simulink model "updated_target_driver_2026_withVariants_MPC_andwlqp"  (R2024b)
settings: Solver=FixedStepDiscrete  StartTime=0.0  StopTime=running_time  FixedStep=dt_s  RelTol=1e-3
values from neighbouring files (symbols this model uses):
  A = gamma_2*gamma_3*Thrust_desired    [force2voltage.m]
  a2_lb = -0.25    [target_driver_setup_2022_Ctrl_V_2_4.m]    (also in target_driver_setup_2022_Ctrl_V_2_4_geometric.m; target_driver_setup_mpc_12msdelay.m; target_driver_setup_mpc_andWLQP.m)
  a2_openloop = 0    [target_driver_setup_2022_Ctrl_V_2_4.m]    (also in target_driver_setup_2022_Ctrl_V_2_4_geometric.m; target_driver_setup_mpc_12msdelay.m; target_driver_setup_mpc_andWLQP.m)
  a2_ub = 0.25    [target_driver_setup_2022_Ctrl_V_2_4.m]    (also in target_driver_setup_2022_Ctrl_V_2_4_geometric.m; target_driver_setup_mpc_12msdelay.m; target_driver_setup_mpc_andWLQP.m)
  att_s = 500    [target_driver_setup_2022_Ctrl_V_2_4.m]    (also in target_driver_setup_2022_Ctrl_V_2_4_geometric.m; target_driver_setup_mpc_12msdelay.m; target_driver_setup_mpc_andWLQP.m)
  b_1_d_desired = [1,0,0]    [target_driver_setup_2022_Ctrl_V_2_4.m]    (also in target_driver_setup_2022_Ctrl_V_2_4_geometric.m; target_driver_setup_mpc_12msdelay.m; target_driver_setup_mpc_andWLQP.m)
  closedloop_flag = 0    [target_driver_setup_2022_Ctrl_V_2_4.m]    (also in target_driver_setup_2022_Ctrl_V_2_4_geometric.m; target_driver_setup_mpc_12msdelay.m; target_driver_setup_mpc_andWLQP.m)
  delay = delay-vicon_sample_cycle/2    [target_driver_setup_2022_Ctrl_V_2_4.m]    (also in target_driver_setup_2022_Ctrl_V_2_4_geometric.m; target_driver_setup_mpc_12msdelay.m; target_driver_setup_mpc_andWLQP.m)
  drv_amp = abs((vleft_p2p-vright_p2p))/2+min(vleft_p2p,vright_p2p)    [Wing_traj_to_Voltage.m]    (also in force2voltage.m; target_driver_setup_2022_Ctrl_V_2_4.m = 150; target_driver_setup_2022_Ctrl_V_2_4_geometric.m = 110; target_driver_setup_mpc_12msdelay.m = 150)
  drv_bias = max_drv_bias    (= 200)    [target_driver_setup_2022_Ctrl_V_2_4.m]    (also in target_driver_setup_2022_Ctrl_V_2_4_geometric.m; target_driver_setup_mpc_12msdelay.m; target_driver_setup_mpc_andWLQP.m)
  drv_pitch_left = vleft_pitch    [Wing_traj_to_Voltage.m]    (also in force2voltage.m = 0; target_driver_setup_2022_Ctrl_V_2_4.m = 9.05; target_driver_setup_2022_Ctrl_V_2_4_geometric.m = 9.05; target_driver_setup_mpc_12msdelay.m = 9.05)
  drv_pitch_right = vright_pitch    [Wing_traj_to_Voltage.m]    (also in force2voltage.m = 0; target_driver_setup_2022_Ctrl_V_2_4.m = 9.05; target_driver_setup_2022_Ctrl_V_2_4_geometric.m = 9.05; target_driver_setup_mpc_12msdelay.m = 9.05)
  drv_roll = (vleft_p2p-vright_p2p)/4    [Wing_traj_to_Voltage.m]    (also in force2voltage.m; target_driver_setup_2022_Ctrl_V_2_4.m = -0.001; target_driver_setup_2022_Ctrl_V_2_4_geometric.m = -0.001; target_driver_setup_mpc_12msdelay.m = -0.001)
  dt_s = 2.0e-4    (= 0.0002)    [target_driver_setup_2022_Ctrl_V_2_4.m]    (also in target_driver_setup_2022_Ctrl_V_2_4_geometric.m; target_driver_setup_mpc_12msdelay.m; target_driver_setup_mpc_andWLQP.m)
  f_fin = f    (= 155)    [target_driver_setup_2022_Ctrl_V_2_4.m]    (also in target_driver_setup_2022_Ctrl_V_2_4_geometric.m; target_driver_setup_mpc_12msdelay.m; target_driver_setup_mpc_andWLQP.m)
  f_int = f    (= 155)    [target_driver_setup_2022_Ctrl_V_2_4.m]    (also in target_driver_setup_2022_Ctrl_V_2_4_geometric.m; target_driver_setup_mpc_12msdelay.m; target_driver_setup_mpc_andWLQP.m)
  g = 9.8    [target_driver_setup_2022_Ctrl_V_2_4.m]    (also in target_driver_setup_2022_Ctrl_V_2_4_geometric.m; target_driver_setup_mpc_12msdelay.m; target_driver_setup_mpc_andWLQP.m; test_full_attitude_mpc.m = 9.81)
  I_moment_vec = [Ixx, Iyy, Izz]    [target_driver_setup_2022_Ctrl_V_2_4.m]    (also in target_driver_setup_2022_Ctrl_V_2_4_geometric.m; target_driver_setup_mpc_12msdelay.m; target_driver_setup_mpc_andWLQP.m)
  k_tau_vec = [k_tau_roll;k_tau_pitch]    [target_driver_setup_2022_Ctrl_V_2_4.m]    (also in target_driver_setup_2022_Ctrl_V_2_4_geometric.m; target_driver_setup_mpc_12msdelay.m; target_driver_setup_mpc_andWLQP.m)
  landing_flag = 0    [target_driver_setup_2022_Ctrl_V_2_4.m]    (also in target_driver_setup_2022_Ctrl_V_2_4_geometric.m; target_driver_setup_mpc_12msdelay.m; target_driver_setup_mpc_andWLQP.m)
  landing_parameter = [start_delay+T,transition_rate, rising_time, falling_time, landing_rising_time, landing_z_decrease, landing_y_decrease, landing_x_decrease]    [target_driver_setup_2022_Ctrl_V_2_4.m]    (also in target_driver_setup_2022_Ctrl_V_2_4_geometric.m; target_driver_setup_mpc_12msdelay.m; target_driver_setup_mpc_andWLQP.m)
  low_bound = -5    [target_driver_setup_2022_Ctrl_V_2_4.m]    (also in target_driver_setup_2022_Ctrl_V_2_4_geometric.m; target_driver_setup_mpc_12msdelay.m = -10; target_driver_setup_mpc_andWLQP.m = -10)
  low_bound_eR = -1.2    [target_driver_setup_2022_Ctrl_V_2_4.m]    (also in target_driver_setup_2022_Ctrl_V_2_4_geometric.m; target_driver_setup_mpc_12msdelay.m; target_driver_setup_mpc_andWLQP.m)
  low_bound_vx = -0.5    [target_driver_setup_2022_Ctrl_V_2_4.m]    (also in target_driver_setup_2022_Ctrl_V_2_4_geometric.m; target_driver_setup_mpc_12msdelay.m; target_driver_setup_mpc_andWLQP.m)
  low_bound_vy = -0.5    [target_driver_setup_2022_Ctrl_V_2_4.m]    (also in target_driver_setup_2022_Ctrl_V_2_4_geometric.m; target_driver_setup_mpc_12msdelay.m; target_driver_setup_mpc_andWLQP.m)
  low_bound_vz = -0.5    [target_driver_setup_2022_Ctrl_V_2_4.m]    (also in target_driver_setup_2022_Ctrl_V_2_4_geometric.m; target_driver_setup_mpc_12msdelay.m; target_driver_setup_mpc_andWLQP.m)
  low_bound_x = -0.1    [target_driver_setup_2022_Ctrl_V_2_4.m]    (also in target_driver_setup_2022_Ctrl_V_2_4_geometric.m; target_driver_setup_mpc_12msdelay.m = -0.6; target_driver_setup_mpc_andWLQP.m = -0.6)
  low_bound_y = -0.06    [target_driver_setup_2022_Ctrl_V_2_4.m]    (also in target_driver_setup_2022_Ctrl_V_2_4_geometric.m; target_driver_setup_mpc_12msdelay.m = -0.6; target_driver_setup_mpc_andWLQP.m = -0.6)
  low_bound_z = -0.04    [target_driver_setup_2022_Ctrl_V_2_4.m]    (also in target_driver_setup_2022_Ctrl_V_2_4_geometric.m; target_driver_setup_mpc_12msdelay.m = -0.1; target_driver_setup_mpc_andWLQP.m = -0.1)
  m = t <= t_zoom    [plot_roll_torque_cmd_vs_actual.m]    (also in plot_roll_torque_cmd_vs_actual_flightlog.m = t >= t0 & t <= t1; target_driver_setup_2022_Ctrl_V_2_4.m = 8.5655e-05; target_driver_setup_2022_Ctrl_V_2_4_geometric.m = 8.5655e-05; target_driver_setup_mpc_12msdelay.m = 8.5655e-05)
  params_vec = [params_opt.delta_1, params_opt.delta_2, params_opt.delta_3,      params_opt.gamma_1, params_opt.gamma_2_1, params_opt.gamma_3,      params_opt.eta, params_opt.nu, params_opt.mu]'    [force2voltage_tuningSandbox.m]    (also in target_driver_setup_2022_Ctrl_V_2_4.m = [params_opt.delta_1, params_opt.delta_2, params_opt.delta_3,; target_driver_setup_2022_Ctrl_V_2_4_geometric.m = [params_opt.delta_1, params_opt.delta_2, params_opt.delta_3,; target_driver_setup_mpc_12msdelay.m = [params_opt.delta_1, params_opt.delta_2, params_opt.delta_3,; target_driver_setup_mpc_andWLQP.m = [params_opt.delta_1, params_opt.delta_2, params_opt.delta_3,)
  phase = 0    [target_driver_setup_2022_Ctrl_V_2_4.m]    (also in target_driver_setup_2022_Ctrl_V_2_4_geometric.m; target_driver_setup_mpc_12msdelay.m; target_driver_setup_mpc_andWLQP.m)
  r_desired = [default_x, default_y,z_desired]    [target_driver_setup_2022_Ctrl_V_2_4.m]    (also in target_driver_setup_2022_Ctrl_V_2_4_geometric.m; target_driver_setup_mpc_12msdelay.m; target_driver_setup_mpc_andWLQP.m)
  roll_offset_angle = 0    [target_driver_setup_2022_Ctrl_V_2_4.m]    (also in target_driver_setup_2022_Ctrl_V_2_4_geometric.m; target_driver_setup_mpc_12msdelay.m; target_driver_setup_mpc_andWLQP.m)
  running_time = start_delay+T    (= 10)    [target_driver_setup_2022_Ctrl_V_2_4.m]    (also in target_driver_setup_2022_Ctrl_V_2_4_geometric.m; target_driver_setup_mpc_12msdelay.m = 0.5; target_driver_setup_mpc_andWLQP.m)
  running_time_control = start_delay_control+T+0.0    (= 10)    [target_driver_setup_2022_Ctrl_V_2_4.m]    (also in target_driver_setup_2022_Ctrl_V_2_4_geometric.m; target_driver_setup_mpc_12msdelay.m = 0.5; target_driver_setup_mpc_andWLQP.m)
  sampling_f = 1/dt_s    (= 5000)    [target_driver_setup_2022_Ctrl_V_2_4.m]    (also in target_driver_setup_2022_Ctrl_V_2_4_geometric.m; target_driver_setup_mpc_12msdelay.m; target_driver_setup_mpc_andWLQP.m)
  start_delay = 0.0    (= 0)    [target_driver_setup_2022_Ctrl_V_2_4.m]    (also in target_driver_setup_2022_Ctrl_V_2_4_geometric.m; target_driver_setup_mpc_12msdelay.m; target_driver_setup_mpc_andWLQP.m)
  start_delay_control = start_delay + ramp_delay    (= 0)    [target_driver_setup_2022_Ctrl_V_2_4.m]    (also in target_driver_setup_2022_Ctrl_V_2_4_geometric.m; target_driver_setup_mpc_12msdelay.m; target_driver_setup_mpc_andWLQP.m)
  T = 10    [target_driver_setup_2022_Ctrl_V_2_4.m]    (also in target_driver_setup_2022_Ctrl_V_2_4_geometric.m; target_driver_setup_mpc_12msdelay.m = 0.5; target_driver_setup_mpc_andWLQP.m; test_full_attitude_mpc.m = T0 + nu(1))
  task_flag = 0    [target_driver_setup_2022_Ctrl_V_2_4.m]    (also in target_driver_setup_2022_Ctrl_V_2_4_geometric.m; target_driver_setup_mpc_12msdelay.m; target_driver_setup_mpc_andWLQP.m)
  task_parameter = [radius_ref, frequency_ref, radius_ratio, lissajous_ratio, lissajous_delta, lissajous_amplitude_ratio,z_radius_ratio]    [target_driver_setup_2022_Ctrl_V_2_4.m]    (also in target_driver_setup_2022_Ctrl_V_2_4_geometric.m; target_driver_setup_mpc_12msdelay.m; target_driver_setup_mpc_andWLQP.m)
  upp_bound = 5    [target_driver_setup_2022_Ctrl_V_2_4.m]    (also in target_driver_setup_2022_Ctrl_V_2_4_geometric.m; target_driver_setup_mpc_12msdelay.m = 10; target_driver_setup_mpc_andWLQP.m = 10)
  upp_bound_eR = 1.2    [target_driver_setup_2022_Ctrl_V_2_4.m]    (also in target_driver_setup_2022_Ctrl_V_2_4_geometric.m; target_driver_setup_mpc_12msdelay.m; target_driver_setup_mpc_andWLQP.m)
  upp_bound_vx = 0.5    [target_driver_setup_2022_Ctrl_V_2_4.m]    (also in target_driver_setup_2022_Ctrl_V_2_4_geometric.m; target_driver_setup_mpc_12msdelay.m; target_driver_setup_mpc_andWLQP.m)
  upp_bound_vy = 0.5    [target_driver_setup_2022_Ctrl_V_2_4.m]    (also in target_driver_setup_2022_Ctrl_V_2_4_geometric.m; target_driver_setup_mpc_12msdelay.m; target_driver_setup_mpc_andWLQP.m)
  upp_bound_vz = 0.5    [target_driver_setup_2022_Ctrl_V_2_4.m]    (also in target_driver_setup_2022_Ctrl_V_2_4_geometric.m; target_driver_setup_mpc_12msdelay.m; target_driver_setup_mpc_andWLQP.m)
  upp_bound_x = 0.1    [target_driver_setup_2022_Ctrl_V_2_4.m]    (also in target_driver_setup_2022_Ctrl_V_2_4_geometric.m; target_driver_setup_mpc_12msdelay.m = 0.6; target_driver_setup_mpc_andWLQP.m = 0.6)
  upp_bound_y = 0.06    [target_driver_setup_2022_Ctrl_V_2_4.m]    (also in target_driver_setup_2022_Ctrl_V_2_4_geometric.m; target_driver_setup_mpc_12msdelay.m = 0.6; target_driver_setup_mpc_andWLQP.m = 0.6)
  upp_bound_z = 0.04    [target_driver_setup_2022_Ctrl_V_2_4.m]    (also in target_driver_setup_2022_Ctrl_V_2_4_geometric.m; target_driver_setup_mpc_12msdelay.m = 0.1; target_driver_setup_mpc_andWLQP.m = 0.1)
  weights_vec = [ws; wds; wpr_xy;wpr_z; wpf; wvr_xy; wvr_z ... (first row only)    [target_driver_setup_2022_Ctrl_V_2_4.m]    (also in target_driver_setup_2022_Ctrl_V_2_4_geometric.m; target_driver_setup_mpc_12msdelay.m; target_driver_setup_mpc_andWLQP.m)
undefined symbols (not defined in the file or in its folder): Com1, ctrl_Ts, DiscIntNeverNeededParam, dspblkCoreblockFVToolHelper, gcbh, left_mapping, left_mapping_F_to_Phi, lp_den, lp_num, none, right_mapping, right_mapping_F_to_Phi, vlp_den, vlp_num
libraries: simulink x18, xpcseriallib x2, cstblocks x1, xpcnilib x1, xpcutilitieslib x1
(part 3 of 6)

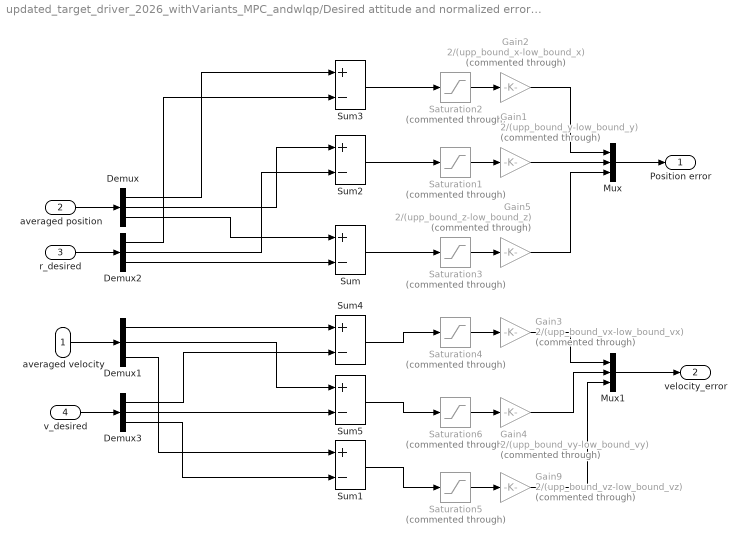
== system updated_target_driver_2026_withVariants_MPC_andwlqp/Desired attitude and normalized error/Variant Subsystem/unsaturated normalized error observation1/saturated normalized altitude error  ==
  averaged velocity : Inport
  averaged position : Inport  Port=2
  "r_desired " : Inport  Port=3
  v_desired : Inport  Port=4
  Demux{,1..3} (4 alike) : Demux  Outputs=3
  Gain1 : Gain  Commented=through  Gain=2/(upp_bound_y-low_bound_y)
  Gain2 : Gain  Commented=through  Gain=2/(upp_bound_x-low_bound_x)
  Gain3 : Gain  Commented=through  Gain=2/(upp_bound_vx-low_bound_vx)
  Gain4 : Gain  Commented=through  Gain=2/(upp_bound_vy-low_bound_vy)
  Gain5 : Gain  Commented=through  Gain=2/(upp_bound_z-low_bound_z)
  Gain9 : Gain  Commented=through  Gain=2/(upp_bound_vz-low_bound_vz)
  Mux : Mux  Inputs=3
  Mux1 : Mux  Inputs=3
  Saturation1 : Saturate  Commented=through  UpperLimit=upp_bound_y  LowerLimit=low_bound_y
  Saturation2 : Saturate  Commented=through  UpperLimit=upp_bound_x  LowerLimit=low_bound_x
  Saturation3 : Saturate  Commented=through  UpperLimit=upp_bound_z  LowerLimit=low_bound_z
  Saturation4 : Saturate  Commented=through  UpperLimit=upp_bound_vx  LowerLimit=low_bound_vx
  Saturation5 : Saturate  Commented=through  UpperLimit=upp_bound_vz  LowerLimit=low_bound_vz
  Saturation6 : Saturate  Commented=through  UpperLimit=upp_bound_vy  LowerLimit=low_bound_vy
  Sum{,1..5} (6 alike) : Sum  Inputs=+-
  Position error : Outport
  velocity_error : Outport  Port=2
  wires:
  Demux2/3 -> Sum/2
  Sum/1 -> Saturation3/1
  Sum1/1 -> Saturation5/1
  Gain5/1 -> Mux/3
  Saturation3/1 -> Gain5/1
  Saturation5/1 -> Gain9/1
  Gain9/1 -> Mux1/3
  Mux1/1 -> velocity_error/1
  averaged velocity/1 -> Demux1/1
  averaged position/1 -> Demux/1
  Demux/3 -> Sum/1
  Demux1/3 -> Sum1/1
  "r_desired "/1 -> Demux2/1
  Saturation1/1 -> Gain1/1
  Sum2/1 -> Saturation1/1
  Demux2/2 -> Sum2/2
  Demux/2 -> Sum2/1
  Sum3/1 -> Saturation2/1
  Saturation2/1 -> Gain2/1
  Demux/1 -> Sum3/1
  Demux2/1 -> Sum3/2
  v_desired/1 -> Demux3/1
  Demux3/3 -> Sum1/2
  Saturation4/1 -> Gain3/1
  Gain3/1 -> Mux1/1
  Sum4/1 -> Saturation4/1
  Demux3/1 -> Sum4/2
  Demux1/1 -> Sum4/1
  Saturation6/1 -> Gain4/1
  Gain4/1 -> Mux1/2
  Sum5/1 -> Saturation6/1
  Demux3/2 -> Sum5/2
  Demux1/2 -> Sum5/1
  Gain2/1 -> Mux/1
  Gain1/1 -> Mux/2
  Mux/1 -> Position error/1

== system updated_target_driver_2026_withVariants_MPC_andwlqp/Observer for averaged system1/Attitude Observer/Geometric Averaging Rotation Matix/Geometric Averaging Rotation M ==
  "Current Rotation " : Inport
  Vicon Update : Inport  Port=2
  "Previous Averaged Rotation " : Inport  Port=3
  Delay1 : Delay  DelayLength=delay(5)  InitialCondition=0
  Delay3 : Delay  DelayLength=delay(2)  InitialCondition=0
  Delay4 : Delay  DelayLength=delay(3)  InitialCondition=0
  Delay5 : Delay  DelayLength=delay(4)  InitialCondition=0
  Delay7 : Delay  DelayLength=delay(6)  InitialCondition=0
  Delay9 : Delay  DelayLength=delay(7)  InitialCondition=0
  "Geometric Average " : MATLAB Function  TreatAsAtomicUnit=on
  Averaged Rotation Matrix : Outport
  wires:
  Delay5/1 -> "Geometric Average "/3(R_prev3)
  Delay4/1 -> "Geometric Average "/2(R_prev2)
  "Geometric Average "/1(Rout) -> Averaged Rotation Matrix/1
  Delay3/1 -> "Geometric Average "/1(R_prev)
  Delay9/1 -> "Geometric Average "/6(R_prev6)
  Delay7/1 -> "Geometric Average "/5(R_prev5)
  Delay1/1 -> "Geometric Average "/4(R_prev4)
  Vicon Update/1 -> "Geometric Average "/8(update)
  "Current Rotation "/1 -> "Geometric Average "/7(R_cur), Delay9/1, Delay7/1, Delay1/1, Delay5/1, Delay4/1, Delay3/1
  "Previous Averaged Rotation "/1 -> "Geometric Average "/9(Rout_prev)

== system updated_target_driver_2026_withVariants_MPC_andwlqp/Observer for averaged system1/Attitude Observer/Geometric derivative in SO(3)/filtered derivative5 ==
  In1 : Inport
  low pass3 : DiscreteTransferFcn  Numerator=lp_num  Denominator=lp_den
  Out1 : Outport
  wires:
  low pass3/1 -> Out1/1
  In1/1 -> low pass3/1

== system updated_target_driver_2026_withVariants_MPC_andwlqp/Variant Subsystem/Experimental/signal generator a3/Bias_Signal ==
  note: time constant = 0.002sec
  QuasiEnable : Inport
  BiasVolts : Inport  Port=2
  AveragedBias : Subsystem
  PreGain : Gain
  Product : Product  RndMeth=Zero
  SIgnalForRamp_binary : Subsystem
  SaturatingRamp : DiscreteIntegrator  gainval=10  SampleTime=-1  LimitOutput=on  UpperSaturationLimit=1  LowerSaturationLimit=0  ICPrevOutput=DiscIntNeverNeededParam  ICPrevScaledInput=DiscIntNeverNeededParam
  BiasD2A : Outport
  wires:
  PreGain/1 -> BiasD2A/1
  BiasVolts/1 -> AveragedBias/1(In1)
  QuasiEnable/1 -> SIgnalForRamp_binary/1(In1)
  SIgnalForRamp_binary/1(Out1) -> SaturatingRamp/1
  SaturatingRamp/1 -> Product/1
  AveragedBias/1(Out1) -> Product/2
  Product/1 -> PreGain/1

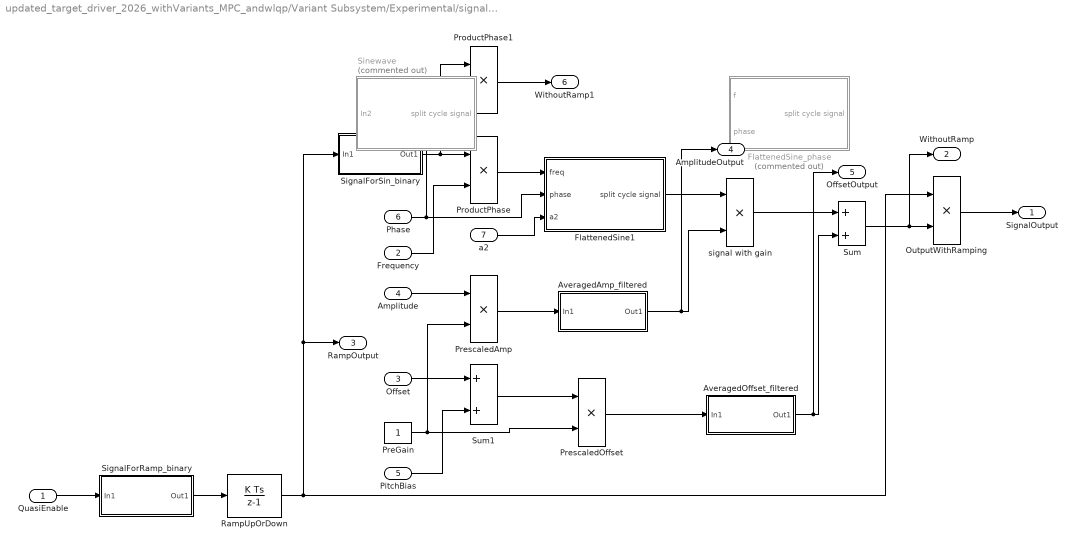
== system updated_target_driver_2026_withVariants_MPC_andwlqp/Variant Subsystem/Experimental/signal generator a3/Drive_Signal ==
  QuasiEnable : Inport
  Frequency : Inport  Port=2
  Offset : Inport  Port=3
  Amplitude : Inport  Port=4
  PitchBias : Inport  Port=5
  Phase : Inport  Port=6
  "a2 " : Inport  Port=7
  AveragedAmp_filtered : Subsystem
  AveragedOffset_filtered : Subsystem
  FlattenedSine1 : Subsystem
  FlattenedSine_phase : Subsystem  Commented=on
  OutputWithRamping : Product  RndMeth=Zero
  PreGain : Constant
  PrescaledAmp : Product  RndMeth=Zero
  PrescaledOffset : Product  RndMeth=Zero
  ProductPhase : Product  RndMeth=Zero
  ProductPhase1 : Product  RndMeth=Zero
  RampUpOrDown : DiscreteIntegrator  gainval=10  SampleTime=-1  LimitOutput=on  UpperSaturationLimit=1  LowerSaturationLimit=0  ICPrevOutput=DiscIntNeverNeededParam  ICPrevScaledInput=DiscIntNeverNeededParam
  SignalForRamp_binary : Subsystem
  SignalForSin_binary : Subsystem
  Sinewave : Subsystem  Commented=on
  Sum : Sum
  Sum1 : Sum
  signal with gain : Product  RndMeth=Zero
  SignalOutput : Outport
  WithoutRamp : Outport  Port=2
  RampOutput : Outport  Port=3
  AmplitudeOutput : Outport  Port=4
  OffsetOutput : Outport  Port=5
  WithoutRamp1 : Outport  Port=6
  wires:
  OutputWithRamping/1 -> SignalOutput/1
  Sum/1 -> WithoutRamp/1, OutputWithRamping/2
  PrescaledOffset/1 -> AveragedOffset_filtered/1(In1)
  AveragedAmp_filtered/1(Out1) -> AmplitudeOutput/1, signal with gain/2
  PrescaledAmp/1 -> AveragedAmp_filtered/1(In1)
  "a2 "/1 -> FlattenedSine1/3(a2)
  ProductPhase/1 -> FlattenedSine1/1(freq)
  ProductPhase1/1 -> WithoutRamp1/1
  Offset/1 -> Sum1/1
  AveragedOffset_filtered/1(Out1) -> OffsetOutput/1, Sum/2
  signal with gain/1 -> Sum/1
  SignalForSin_binary/1(Out1) -> ProductPhase1/1, ProductPhase/1
  Amplitude/1 -> PrescaledAmp/1
  Sum1/1 -> PrescaledOffset/1
  Frequency/1 -> ProductPhase/2
  PreGain/1 -> PrescaledAmp/2, PrescaledOffset/2
  FlattenedSine1/1(split cycle signal) -> signal with gain/1
  QuasiEnable/1 -> SignalForRamp_binary/1(In1)
  SignalForRamp_binary/1(Out1) -> RampUpOrDown/1
  Phase/1 -> ProductPhase1/2, FlattenedSine1/2(phase)
  PitchBias/1 -> Sum1/2
  RampUpOrDown/1 -> SignalForSin_binary/1(In1), RampOutput/1, OutputWithRamping/1

== system updated_target_driver_2026_withVariants_MPC_andwlqp/Variant Subsystem/Experimental/signal generator a3/Drive_Signal1 ==
  QuasiEnable : Inport
  Frequency : Inport  Port=2
  Offset : Inport  Port=3
  Amplitude : Inport  Port=4
  PitchBias : Inport  Port=5
  a2 : Inport  Port=6
  AveragedAmp_filtered : Subsystem
  AveragedOffset_filtered : Subsystem
  FlattenedSine1 : Subsystem
  OutputWithRamping : Product  RndMeth=Zero
  PreGain : Constant
  PrescaledAmp : Product  RndMeth=Zero
  PrescaledOffset : Product  RndMeth=Zero
  ProductPhase : Product  RndMeth=Zero
  RampUpOrDown : DiscreteIntegrator  gainval=10  SampleTime=-1  LimitOutput=on  UpperSaturationLimit=1  LowerSaturationLimit=0  ICPrevOutput=DiscIntNeverNeededParam  ICPrevScaledInput=DiscIntNeverNeededParam
  SignalForRamp_binary : Subsystem
  SignalForSin_binary : Subsystem
  Sine Wave : Subsystem  Commented=on
  Sum : Sum
  Sum1 : Sum
  signal with gain : Product  RndMeth=Zero
  SignalOutput : Outport
  WithoutRamp : Outport  Port=2
  RampOutput : Outport  Port=3
  AmplitudeOutput : Outport  Port=4
  OffsetOutput : Outport  Port=5
  wires:
  PrescaledAmp/1 -> AveragedAmp_filtered/1(In1)
  Sum/1 -> OutputWithRamping/2, WithoutRamp/1
  RampUpOrDown/1 -> RampOutput/1, OutputWithRamping/1, SignalForSin_binary/1(In1)
  QuasiEnable/1 -> SignalForRamp_binary/1(In1)
  SignalForRamp_binary/1(Out1) -> RampUpOrDown/1
  signal with gain/1 -> Sum/1
  Frequency/1 -> ProductPhase/2
  SignalForSin_binary/1(Out1) -> ProductPhase/1
  AveragedOffset_filtered/1(Out1) -> Sum/2, OffsetOutput/1
  PrescaledOffset/1 -> AveragedOffset_filtered/1(In1)
  PreGain/1 -> PrescaledAmp/2, PrescaledOffset/2
  OutputWithRamping/1 -> SignalOutput/1
  AveragedAmp_filtered/1(Out1) -> signal with gain/2, AmplitudeOutput/1
  Sum1/1 -> PrescaledOffset/1
  Offset/1 -> Sum1/1
  PitchBias/1 -> Sum1/2
  Amplitude/1 -> PrescaledAmp/1
  ProductPhase/1 -> FlattenedSine1/1(freq)
  FlattenedSine1/1(split cycle signal) -> signal with gain/1
  a2/1 -> FlattenedSine1/2(a2)

== system updated_target_driver_2026_withVariants_MPC_andwlqp/Variant Subsystem/Experimental/signal generator a3/SignalSaturationLimit ==
  BiasMax : Inport
  SignalRaw : Inport  Port=2
  GainBias : Gain
  MaxOf : MinMax  Function=max  Inputs=2
  MinOf : MinMax  Inputs=2
  ground : Constant
  SignalSatd : Outport
  wires:
  BiasMax/1 -> GainBias/1
  SignalRaw/1 -> MinOf/2
  MinOf/1 -> MaxOf/1
  MaxOf/1 -> SignalSatd/1
  GainBias/1 -> MinOf/1
  ground/1 -> MaxOf/2

== system updated_target_driver_2026_withVariants_MPC_andwlqp/Variant Subsystem/Experimental/signal generator a3/SignalSaturationLimit1 ==
  BiasMax : Inport
  SignalRaw : Inport  Port=2
  GainBias : Gain
  MaxOf : MinMax  Function=max  Inputs=2
  MinOf : MinMax  Inputs=2
  ground : Constant
  SignalSatd : Outport
  wires:
  BiasMax/1 -> GainBias/1
  SignalRaw/1 -> MinOf/2
  MinOf/1 -> MaxOf/1
  MaxOf/1 -> SignalSatd/1
  GainBias/1 -> MinOf/1
  ground/1 -> MaxOf/2

== system updated_target_driver_2026_withVariants_MPC_andwlqp/Variant Subsystem/Simulation/signal generator a3/Bias_Signal ==
  note: time constant = 0.002sec
  QuasiEnable : Inport
  BiasVolts : Inport  Port=2
  AveragedBias : Subsystem
  PreGain : Gain
  Product : Product  RndMeth=Zero
  SIgnalForRamp_binary : Subsystem
  SaturatingRamp : DiscreteIntegrator  Commented=through  gainval=10  SampleTime=-1  LimitOutput=on  UpperSaturationLimit=1  LowerSaturationLimit=0  ICPrevOutput=DiscIntNeverNeededParam  ICPrevScaledInput=DiscIntNeverNeededParam
  BiasD2A : Outport
  wires:
  PreGain/1 -> BiasD2A/1
  BiasVolts/1 -> AveragedBias/1(In1)
  QuasiEnable/1 -> SIgnalForRamp_binary/1(In1)
  SIgnalForRamp_binary/1(Out1) -> SaturatingRamp/1
  SaturatingRamp/1 -> Product/1
  AveragedBias/1(Out1) -> Product/2
  Product/1 -> PreGain/1

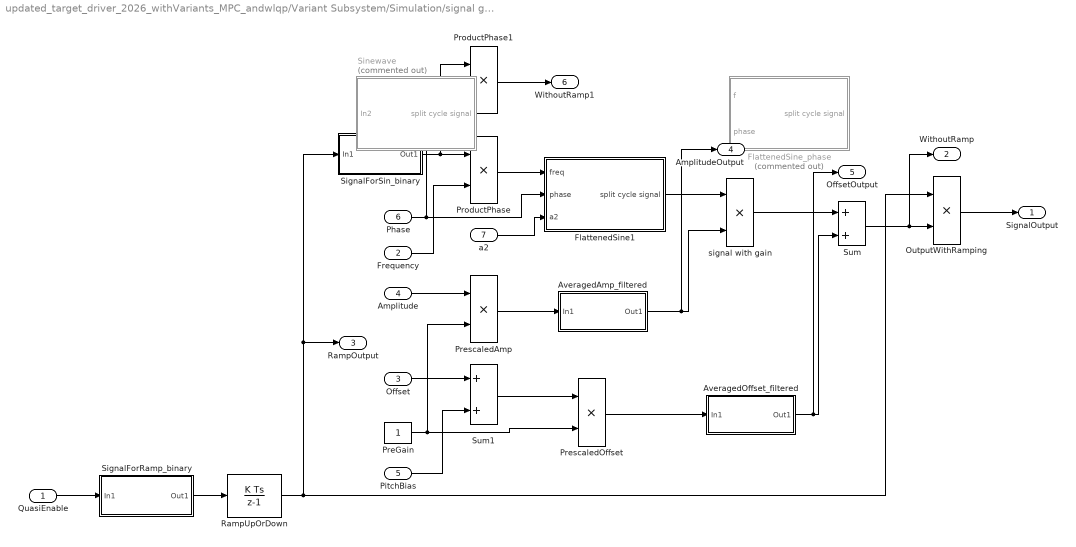
== system updated_target_driver_2026_withVariants_MPC_andwlqp/Variant Subsystem/Simulation/signal generator a3/Drive_Signal ==
  QuasiEnable : Inport
  Frequency : Inport  Port=2
  Offset : Inport  Port=3
  Amplitude : Inport  Port=4
  PitchBias : Inport  Port=5
  Phase : Inport  Port=6
  "a2 " : Inport  Port=7
  AveragedAmp_filtered : Subsystem
  AveragedOffset_filtered : Subsystem
  FlattenedSine1 : Subsystem
  FlattenedSine_phase : Subsystem  Commented=on
  OutputWithRamping : Product  RndMeth=Zero
  PreGain : Constant
  PrescaledAmp : Product  RndMeth=Zero
  PrescaledOffset : Product  RndMeth=Zero
  ProductPhase : Product  RndMeth=Zero
  ProductPhase1 : Product  RndMeth=Zero
  RampUpOrDown : DiscreteIntegrator  gainval=10  SampleTime=-1  LimitOutput=on  UpperSaturationLimit=1  LowerSaturationLimit=0  ICPrevOutput=DiscIntNeverNeededParam  ICPrevScaledInput=DiscIntNeverNeededParam
  SignalForRamp_binary : Subsystem
  SignalForSin_binary : Subsystem
  Sinewave : Subsystem  Commented=on
  Sum : Sum
  Sum1 : Sum
  signal with gain : Product  RndMeth=Zero
  SignalOutput : Outport
  WithoutRamp : Outport  Port=2
  RampOutput : Outport  Port=3
  AmplitudeOutput : Outport  Port=4
  OffsetOutput : Outport  Port=5
  WithoutRamp1 : Outport  Port=6
  wires:
  OutputWithRamping/1 -> SignalOutput/1
  Sum/1 -> WithoutRamp/1, OutputWithRamping/2
  PrescaledOffset/1 -> AveragedOffset_filtered/1(In1)
  AveragedAmp_filtered/1(Out1) -> AmplitudeOutput/1, signal with gain/2
  PrescaledAmp/1 -> AveragedAmp_filtered/1(In1)
  "a2 "/1 -> FlattenedSine1/3(a2)
  ProductPhase/1 -> FlattenedSine1/1(freq)
  ProductPhase1/1 -> WithoutRamp1/1
  Offset/1 -> Sum1/1
  AveragedOffset_filtered/1(Out1) -> OffsetOutput/1, Sum/2
  signal with gain/1 -> Sum/1
  SignalForSin_binary/1(Out1) -> ProductPhase1/1, ProductPhase/1
  Amplitude/1 -> PrescaledAmp/1
  Sum1/1 -> PrescaledOffset/1
  Frequency/1 -> ProductPhase/2
  PreGain/1 -> PrescaledAmp/2, PrescaledOffset/2
  FlattenedSine1/1(split cycle signal) -> signal with gain/1
  QuasiEnable/1 -> SignalForRamp_binary/1(In1)
  SignalForRamp_binary/1(Out1) -> RampUpOrDown/1
  Phase/1 -> ProductPhase1/2, FlattenedSine1/2(phase)
  PitchBias/1 -> Sum1/2
  RampUpOrDown/1 -> SignalForSin_binary/1(In1), RampOutput/1, OutputWithRamping/1

== system updated_target_driver_2026_withVariants_MPC_andwlqp/Variant Subsystem/Simulation/signal generator a3/Drive_Signal1 ==
  QuasiEnable : Inport
  Frequency : Inport  Port=2
  Offset : Inport  Port=3
  Amplitude : Inport  Port=4
  PitchBias : Inport  Port=5
  a2 : Inport  Port=6
  AveragedAmp_filtered : Subsystem
  AveragedOffset_filtered : Subsystem
  FlattenedSine1 : Subsystem
  OutputWithRamping : Product  RndMeth=Zero
  PreGain : Constant
  PrescaledAmp : Product  RndMeth=Zero
  PrescaledOffset : Product  RndMeth=Zero
  ProductPhase : Product  RndMeth=Zero
  RampUpOrDown : DiscreteIntegrator  gainval=10  SampleTime=-1  LimitOutput=on  UpperSaturationLimit=1  LowerSaturationLimit=0  ICPrevOutput=DiscIntNeverNeededParam  ICPrevScaledInput=DiscIntNeverNeededParam
  SignalForRamp_binary : Subsystem
  SignalForSin_binary : Subsystem
  Sine Wave : Subsystem  Commented=on
  Sum : Sum
  Sum1 : Sum
  signal with gain : Product  RndMeth=Zero
  SignalOutput : Outport
  WithoutRamp : Outport  Port=2
  RampOutput : Outport  Port=3
  AmplitudeOutput : Outport  Port=4
  OffsetOutput : Outport  Port=5
  wires:
  PrescaledAmp/1 -> AveragedAmp_filtered/1(In1)
  Sum/1 -> OutputWithRamping/2, WithoutRamp/1
  RampUpOrDown/1 -> RampOutput/1, OutputWithRamping/1, SignalForSin_binary/1(In1)
  QuasiEnable/1 -> SignalForRamp_binary/1(In1)
  SignalForRamp_binary/1(Out1) -> RampUpOrDown/1
  signal with gain/1 -> Sum/1
  Frequency/1 -> ProductPhase/2
  SignalForSin_binary/1(Out1) -> ProductPhase/1
  AveragedOffset_filtered/1(Out1) -> Sum/2, OffsetOutput/1
  PrescaledOffset/1 -> AveragedOffset_filtered/1(In1)
  PreGain/1 -> PrescaledAmp/2, PrescaledOffset/2
  OutputWithRamping/1 -> SignalOutput/1
  AveragedAmp_filtered/1(Out1) -> signal with gain/2, AmplitudeOutput/1
  Sum1/1 -> PrescaledOffset/1
  Offset/1 -> Sum1/1
  PitchBias/1 -> Sum1/2
  Amplitude/1 -> PrescaledAmp/1
  ProductPhase/1 -> FlattenedSine1/1(freq)
  FlattenedSine1/1(split cycle signal) -> signal with gain/1
  a2/1 -> FlattenedSine1/2(a2)

== system updated_target_driver_2026_withVariants_MPC_andwlqp/Variant Subsystem/Simulation/signal generator a3/SignalSaturationLimit ==
  BiasMax : Inport
  SignalRaw : Inport  Port=2
  GainBias : Gain
  MaxOf : MinMax  Function=max  Inputs=2
  MinOf : MinMax  Inputs=2
  ground : Constant
  SignalSatd : Outport
  wires:
  BiasMax/1 -> GainBias/1
  SignalRaw/1 -> MinOf/2
  MinOf/1 -> MaxOf/1
  MaxOf/1 -> SignalSatd/1
  GainBias/1 -> MinOf/1
  ground/1 -> MaxOf/2

== system updated_target_driver_2026_withVariants_MPC_andwlqp/Variant Subsystem/Simulation/signal generator a3/SignalSaturationLimit1 ==
  BiasMax : Inport
  SignalRaw : Inport  Port=2
  GainBias : Gain
  MaxOf : MinMax  Function=max  Inputs=2
  MinOf : MinMax  Inputs=2
  ground : Constant
  SignalSatd : Outport
  wires:
  BiasMax/1 -> GainBias/1
  SignalRaw/1 -> MinOf/2
  MinOf/1 -> MaxOf/1
  MaxOf/1 -> SignalSatd/1
  GainBias/1 -> MinOf/1
  ground/1 -> MaxOf/2

== system updated_target_driver_2026_withVariants_MPC_andwlqp/Vicon Post Processing1/Vicon Validity check/Variant Subsystem1/Experimental ==
  In1 : Inport
  Out1 : Outport
  wires:
  In1/1 -> Out1/1

== system updated_target_driver_2026_withVariants_MPC_andwlqp/Vicon Post Processing1/Vicon Validity check/Variant Subsystem1/Simulation ==
  In1 : Inport
  Discrete Pulse Generator : DiscretePulseGenerator  Period=5  SampleTime=dt_s
  Terminator : Terminator
  Out1 : Outport
  wires:
  Discrete Pulse Generator/1 -> Out1/1
  In1/1 -> Terminator/1

== system updated_target_driver_2026_withVariants_MPC_andwlqp/Variant Subsystem/Experimental/signal generator a3/Bias_Signal/AveragedBias ==
  note: To avoid having signal "jump",
      | we want SMOOTH transitions
      | in frequency (i.e., a weighted sum
      | of current freq and freq some delta t ago)
  note: time constant = 0.002sec
  In1 : Inport
  Discrete Transfer Fcn : DiscreteTransferFcn  Numerator=[0.05]  Denominator=[1 -.95]
  Out1 : Outport
  wires:
  In1/1 -> Discrete Transfer Fcn/1
  Discrete Transfer Fcn/1 -> Out1/1

== system updated_target_driver_2026_withVariants_MPC_andwlqp/Variant Subsystem/Experimental/signal generator a3/Bias_Signal/SIgnalForRamp_binary ==
  note: Should output 1 or -1,
      | so signal ramps UP to 1
      | or DOWN to 0.
  In1 : Inport
  Add : Sum  Inputs=+-
  Compare To Zero : simulink/Logic and Bit Operations/Compare To Zero  relop=>  OutDataTypeStr=uint8  ZeroCross=off
  Constant : Constant
  Data Type Conversion : DataTypeConversion  OutDataTypeStr=double  SaturateOnIntegerOverflow=off  RndMeth=Floor
  Gain : Gain  Gain=2
  Out1 : Outport
  wires:
  In1/1 -> Compare To Zero/1
  Compare To Zero/1 -> Data Type Conversion/1
  Gain/1 -> Add/1
  Constant/1 -> Add/2
  Add/1 -> Out1/1
  Data Type Conversion/1 -> Gain/1

== system updated_target_driver_2026_withVariants_MPC_andwlqp/Variant Subsystem/Experimental/signal generator a3/Drive_Signal/AveragedAmp_filtered ==
  note: To avoid having signal "jump",
      | we want SMOOTH transitions
      | in frequency (i.e., a weighted sum
      | of current freq and freq some delta t ago)
  note: time constant 0.002sec
      | for 10kHz samping
  In1 : Inport
  Discrete Transfer Fcn : DiscreteTransferFcn  Numerator=[0.05]  Denominator=[1 -.95]
  Out1 : Outport
  wires:
  In1/1 -> Discrete Transfer Fcn/1
  Discrete Transfer Fcn/1 -> Out1/1

== system updated_target_driver_2026_withVariants_MPC_andwlqp/Variant Subsystem/Experimental/signal generator a3/Drive_Signal/AveragedOffset_filtered ==
  note: To avoid having signal "jump",
      | we want SMOOTH transitions
      | in frequency (i.e., a weighted sum
      | of current freq and freq some delta t ago)
  note: c
  note: time constant 0.02sec
      | for 10kHz samping
  In1 : Inport
  Discrete Transfer Fcn : DiscreteTransferFcn  Numerator=[0.05]  Denominator=[1 -.95]
  Out1 : Outport
  wires:
  In1/1 -> Discrete Transfer Fcn/1
  Discrete Transfer Fcn/1 -> Out1/1

== system updated_target_driver_2026_withVariants_MPC_andwlqp/Variant Subsystem/Experimental/signal generator a3/Drive_Signal/FlattenedSine1 ==
  freq : Inport
  phase : Inport  Port=2
  a2 : Inport  Port=3
  0.1 : Gain  Gain=0.1
  1.1 : Gain  Gain=1.1
  2f : Gain  Gain=2
  2pi : Gain  Gain=2*pi
  3f : Gain  Gain=3
  Add : Sum  Inputs=+++
  Add1 : Sum
  Amplitude Correction : Subsystem  Commented=on
  AveragedAmp_filtered : Subsystem
  Product : Product
  first harmonic : Trigonometry  OutputSignalType=real
  integrate(omega*t) : DiscreteIntegrator  SampleTime=-1  ICPrevOutput=DiscIntNeverNeededParam  ICPrevScaledInput=DiscIntNeverNeededParam
  second harmonic : Trigonometry  OutputSignalType=real
  third harmonic : Trigonometry  OutputSignalType=real
  split cycle signal : Outport
  wires:
  freq/1 -> 2pi/1
  2pi/1 -> integrate(omega*t)/1
  3f/1 -> third harmonic/1
  first harmonic/1 -> 1.1/1
  third harmonic/1 -> 0.1/1
  1.1/1 -> Add/1
  Add1/1 -> first harmonic/1, 2f/1, 3f/1
  integrate(omega*t)/1 -> Add1/1
  phase/1 -> Add1/2
  2f/1 -> second harmonic/1
  0.1/1 -> Add/2
  Product/1 -> Add/3
  second harmonic/1 -> Product/1
  Add/1 -> split cycle signal/1
  a2/1 -> AveragedAmp_filtered/1(In1)
  AveragedAmp_filtered/1(Out1) -> Product/2

== system updated_target_driver_2026_withVariants_MPC_andwlqp/Variant Subsystem/Experimental/signal generator a3/Drive_Signal/FlattenedSine_phase ==
  f : Inport
  phase : Inport  Port=2
  0.1 : Gain  Gain=0.1
  1.1 : Gain  Gain=1.1
  2pi : Gain  Gain=2*pi
  3f : Gain  Gain=3
  Add : Sum
  Sum : Sum  Inputs=|++
  first harmonic : Trigonometry  OutputSignalType=real
  integrate(omega*t) : DiscreteIntegrator  SampleTime=-1  ICPrevOutput=DiscIntNeverNeededParam  ICPrevScaledInput=DiscIntNeverNeededParam
  pi/180 : Gain  Gain=pi/180
  third harmonic : Trigonometry  OutputSignalType=real
  split cycle signal : Outport
  wires:
  f/1 -> 2pi/1
  2pi/1 -> integrate(omega*t)/1
  3f/1 -> third harmonic/1
  first harmonic/1 -> 1.1/1
  third harmonic/1 -> 0.1/1
  1.1/1 -> Add/1
  0.1/1 -> Add/2
  Add/1 -> split cycle signal/1
  Sum/1 -> first harmonic/1, 3f/1
  pi/180/1 -> Sum/2
  integrate(omega*t)/1 -> Sum/1
  phase/1 -> pi/180/1

== system updated_target_driver_2026_withVariants_MPC_andwlqp/Variant Subsystem/Experimental/signal generator a3/Drive_Signal/SignalForRamp_binary ==
  note: Should output 1 or -1,
      | so signal ramps UP to 1
      | or DOWN to 0.
  In1 : Inport
  Add : Sum  Inputs=+-
  Compare To Zero : simulink/Logic and Bit Operations/Compare To Zero  relop=>  OutDataTypeStr=uint8  ZeroCross=off
  Constant : Constant
  Data Type Conversion : DataTypeConversion  OutDataTypeStr=double  SaturateOnIntegerOverflow=off  RndMeth=Floor
  Gain : Gain  Gain=2
  Out1 : Outport
  wires:
  In1/1 -> Compare To Zero/1
  Compare To Zero/1 -> Data Type Conversion/1
  Gain/1 -> Add/1
  Constant/1 -> Add/2
  Add/1 -> Out1/1
  Data Type Conversion/1 -> Gain/1

== system updated_target_driver_2026_withVariants_MPC_andwlqp/Variant Subsystem/Experimental/signal generator a3/Drive_Signal/SignalForSin_binary ==
  note: We want this to stay "high" for 1
      | second after the actual "enable"
      | is turned off...
  In1 : Inport
  Compare To Zero : simulink/Logic and Bit Operations/Compare To Zero  relop=>  OutDataTypeStr=uint8  ZeroCross=off
  Data Type Conversion : DataTypeConversion  OutDataTypeStr=double  SaturateOnIntegerOverflow=off  RndMeth=Floor
  Out1 : Outport
  wires:
  In1/1 -> Compare To Zero/1
  Compare To Zero/1 -> Data Type Conversion/1
  Data Type Conversion/1 -> Out1/1

== system updated_target_driver_2026_withVariants_MPC_andwlqp/Variant Subsystem/Experimental/signal generator a3/Drive_Signal/Sinewave ==
  In2 : Inport
  2pi : Gain  Gain=2*pi
  first harmonic : Trigonometry  OutputSignalType=real
  integrate(omega*t) : DiscreteIntegrator  SampleTime=-1  ICPrevOutput=DiscIntNeverNeededParam  ICPrevScaledInput=DiscIntNeverNeededParam
  split cycle signal : Outport
  wires:
  In2/1 -> 2pi/1
  2pi/1 -> integrate(omega*t)/1
  integrate(omega*t)/1 -> first harmonic/1
  first harmonic/1 -> split cycle signal/1

== system updated_target_driver_2026_withVariants_MPC_andwlqp/Variant Subsystem/Experimental/signal generator a3/Drive_Signal1/AveragedAmp_filtered ==
  note: To avoid having signal "jump",
      | we want SMOOTH transitions
      | in frequency (i.e., a weighted sum
      | of current freq and freq some delta t ago)
  note: time constant 0.002sec
      | for 10kHz samping
  In1 : Inport
  Discrete Transfer Fcn : DiscreteTransferFcn  Numerator=[0.05]  Denominator=[1 -.95]
  Out1 : Outport
  wires:
  In1/1 -> Discrete Transfer Fcn/1
  Discrete Transfer Fcn/1 -> Out1/1

== system updated_target_driver_2026_withVariants_MPC_andwlqp/Variant Subsystem/Experimental/signal generator a3/Drive_Signal1/AveragedOffset_filtered ==
  note: To avoid having signal "jump",
      | we want SMOOTH transitions
      | in frequency (i.e., a weighted sum
      | of current freq and freq some delta t ago)
  note: c
  note: time constant 0.02sec
      | for 10kHz samping
  In1 : Inport
  Discrete Transfer Fcn : DiscreteTransferFcn  LoadFcn=dspblkCoreblockFVToolHelper(gcbh,'load');  Numerator=[0.05]  Denominator=[1 -.95]
      settings: CopyFcn=dspblkCoreblockFVToolHelper(gcbh,'copy');  DeleteFcn=dspblkCoreblockFVToolHelper(gcbh,'close');  ModelCloseFcn=dspblkCoreblockFVToolHelper(gcbh,'close');  PreSaveFcn=dspblkCoreblockFVToolHelper(gcbh,'presave');  PostSaveFcn=dspblkCoreblockFVToolHelper(gcbh,'postsave');  CloseFcn=dspblkCoreblockFVToolHelper(gcbh,'close');
  Out1 : Outport
  wires:
  In1/1 -> Discrete Transfer Fcn/1
  Discrete Transfer Fcn/1 -> Out1/1

== system updated_target_driver_2026_withVariants_MPC_andwlqp/Variant Subsystem/Experimental/signal generator a3/Drive_Signal1/FlattenedSine1 ==
  freq : Inport
  a2 : Inport  Port=2
  0.1 : Gain  Gain=0.1
  0.2 : Gain  Gain=-1
  1.1 : Gain  Gain=1.1
  2f : Gain  Gain=2
  2pi : Gain  Gain=2*pi
  3f : Gain  Gain=3
  Add : Sum  Inputs=+++
  Amplitude Correction : Subsystem  Commented=on
  AveragedAmp_filtered : Subsystem
  Product : Product
  first harmonic : Trigonometry  OutputSignalType=real
  integrate(omega*t) : DiscreteIntegrator  SampleTime=-1  ICPrevOutput=DiscIntNeverNeededParam  ICPrevScaledInput=DiscIntNeverNeededParam
  second harmonic : Trigonometry  OutputSignalType=real
  third harmonic : Trigonometry  OutputSignalType=real
  split cycle signal : Outport
  wires:
  freq/1 -> 2pi/1
  2pi/1 -> integrate(omega*t)/1
  3f/1 -> third harmonic/1
  first harmonic/1 -> 1.1/1
  third harmonic/1 -> 0.1/1
  1.1/1 -> Add/1
  integrate(omega*t)/1 -> first harmonic/1, 2f/1, 3f/1
  2f/1 -> second harmonic/1
  0.1/1 -> Add/2
  Product/1 -> Add/3
  second harmonic/1 -> Product/1
  0.2/1 -> Product/2
  Add/1 -> split cycle signal/1
  a2/1 -> AveragedAmp_filtered/1(In1)
  AveragedAmp_filtered/1(Out1) -> 0.2/1

== system updated_target_driver_2026_withVariants_MPC_andwlqp/Variant Subsystem/Experimental/signal generator a3/Drive_Signal1/SignalForRamp_binary ==
  note: Should output 1 or -1,
      | so signal ramps UP to 1
      | or DOWN to 0.
  In1 : Inport
  Add : Sum  Inputs=+-
  Compare To Zero : simulink/Logic and Bit Operations/Compare To Zero  relop=>  OutDataTypeStr=uint8  ZeroCross=off
  Constant : Constant
  Data Type Conversion : DataTypeConversion  OutDataTypeStr=double  SaturateOnIntegerOverflow=off  RndMeth=Floor
  Gain : Gain  Gain=2
  Out1 : Outport
  wires:
  In1/1 -> Compare To Zero/1
  Compare To Zero/1 -> Data Type Conversion/1
  Gain/1 -> Add/1
  Constant/1 -> Add/2
  Add/1 -> Out1/1
  Data Type Conversion/1 -> Gain/1

== system updated_target_driver_2026_withVariants_MPC_andwlqp/Variant Subsystem/Experimental/signal generator a3/Drive_Signal1/SignalForSin_binary ==
  note: We want this to stay "high" for 1
      | second after the actual "enable"
      | is turned off...
  In1 : Inport
  Compare To Zero : simulink/Logic and Bit Operations/Compare To Zero  relop=>  OutDataTypeStr=uint8  ZeroCross=off
  Data Type Conversion : DataTypeConversion  OutDataTypeStr=double  SaturateOnIntegerOverflow=off  RndMeth=Floor
  Out1 : Outport
  wires:
  In1/1 -> Compare To Zero/1
  Compare To Zero/1 -> Data Type Conversion/1
  Data Type Conversion/1 -> Out1/1

== system updated_target_driver_2026_withVariants_MPC_andwlqp/Variant Subsystem/Experimental/signal generator a3/Drive_Signal1/Sine Wave ==
  In2 : Inport
  2pi : Gain  Gain=2*pi
  first harmonic : Trigonometry  OutputSignalType=real
  integrate(omega*t) : DiscreteIntegrator  SampleTime=-1  ICPrevOutput=DiscIntNeverNeededParam  ICPrevScaledInput=DiscIntNeverNeededParam
  split cycle signal : Outport
  wires:
  In2/1 -> 2pi/1
  2pi/1 -> integrate(omega*t)/1
  integrate(omega*t)/1 -> first harmonic/1
  first harmonic/1 -> split cycle signal/1

== system updated_target_driver_2026_withVariants_MPC_andwlqp/Variant Subsystem/Simulation/signal generator a3/Bias_Signal/AveragedBias ==
  note: To avoid having signal "jump",
      | we want SMOOTH transitions
      | in frequency (i.e., a weighted sum
      | of current freq and freq some delta t ago)
  note: time constant = 0.002sec
  In1 : Inport
  Discrete Transfer Fcn : DiscreteTransferFcn  LoadFcn=dspblkCoreblockFVToolHelper(gcbh,'load');  Numerator=[0.05]  Denominator=[1 -.95]
      settings: CopyFcn=dspblkCoreblockFVToolHelper(gcbh,'copy');  DeleteFcn=dspblkCoreblockFVToolHelper(gcbh,'close');  ModelCloseFcn=dspblkCoreblockFVToolHelper(gcbh,'close');  PreSaveFcn=dspblkCoreblockFVToolHelper(gcbh,'presave');  PostSaveFcn=dspblkCoreblockFVToolHelper(gcbh,'postsave');  CloseFcn=dspblkCoreblockFVToolHelper(gcbh,'close');
  Out1 : Outport
  wires:
  In1/1 -> Discrete Transfer Fcn/1
  Discrete Transfer Fcn/1 -> Out1/1

== system updated_target_driver_2026_withVariants_MPC_andwlqp/Variant Subsystem/Simulation/signal generator a3/Bias_Signal/SIgnalForRamp_binary ==
  note: Should output 1 or -1,
      | so signal ramps UP to 1
      | or DOWN to 0.
  In1 : Inport
  Add : Sum  Inputs=+-
  Compare To Zero : simulink/Logic and Bit Operations/Compare To Zero  relop=>  OutDataTypeStr=uint8  ZeroCross=off
  Constant : Constant
  Data Type Conversion : DataTypeConversion  OutDataTypeStr=double  SaturateOnIntegerOverflow=off  RndMeth=Floor
  Gain : Gain  Gain=2
  Out1 : Outport
  wires:
  In1/1 -> Compare To Zero/1
  Compare To Zero/1 -> Data Type Conversion/1
  Gain/1 -> Add/1
  Constant/1 -> Add/2
  Add/1 -> Out1/1
  Data Type Conversion/1 -> Gain/1

== system updated_target_driver_2026_withVariants_MPC_andwlqp/Variant Subsystem/Simulation/signal generator a3/Drive_Signal/AveragedAmp_filtered ==
  note: To avoid having signal "jump",
      | we want SMOOTH transitions
      | in frequency (i.e., a weighted sum
      | of current freq and freq some delta t ago)
  note: time constant 0.002sec
      | for 10kHz samping
  In1 : Inport
  Discrete Transfer Fcn : DiscreteTransferFcn  LoadFcn=dspblkCoreblockFVToolHelper(gcbh,'load');  Numerator=[0.05]  Denominator=[1 -.95]
      settings: CopyFcn=dspblkCoreblockFVToolHelper(gcbh,'copy');  DeleteFcn=dspblkCoreblockFVToolHelper(gcbh,'close');  ModelCloseFcn=dspblkCoreblockFVToolHelper(gcbh,'close');  PreSaveFcn=dspblkCoreblockFVToolHelper(gcbh,'presave');  PostSaveFcn=dspblkCoreblockFVToolHelper(gcbh,'postsave');  CloseFcn=dspblkCoreblockFVToolHelper(gcbh,'close');
  Discrete Transfer Fcn2 : DiscreteTransferFcn  LoadFcn=dspblkCoreblockFVToolHelper(gcbh,'load');  Numerator=[0.37152]  Denominator=[1 -.62848]
      settings: CopyFcn=dspblkCoreblockFVToolHelper(gcbh,'copy');  DeleteFcn=dspblkCoreblockFVToolHelper(gcbh,'close');  ModelCloseFcn=dspblkCoreblockFVToolHelper(gcbh,'close');  PreSaveFcn=dspblkCoreblockFVToolHelper(gcbh,'presave');  PostSaveFcn=dspblkCoreblockFVToolHelper(gcbh,'postsave');  CloseFcn=dspblkCoreblockFVToolHelper(gcbh,'close');
  Out1 : Outport
  wires:
  In1/1 -> Discrete Transfer Fcn2/1
  Discrete Transfer Fcn2/1 -> Out1/1

== system updated_target_driver_2026_withVariants_MPC_andwlqp/Variant Subsystem/Simulation/signal generator a3/Drive_Signal/AveragedOffset_filtered ==
  note: To avoid having signal "jump",
      | we want SMOOTH transitions
      | in frequency (i.e., a weighted sum
      | of current freq and freq some delta t ago)
  note: time constant 0.02sec
      | for 10kHz samping
  In1 : Inport
  Discrete Transfer Fcn : DiscreteTransferFcn  LoadFcn=dspblkCoreblockFVToolHelper(gcbh,'load');  Numerator=[0.05]  Denominator=[1 -.95]
      settings: CopyFcn=dspblkCoreblockFVToolHelper(gcbh,'copy');  DeleteFcn=dspblkCoreblockFVToolHelper(gcbh,'close');  ModelCloseFcn=dspblkCoreblockFVToolHelper(gcbh,'close');  PreSaveFcn=dspblkCoreblockFVToolHelper(gcbh,'presave');  PostSaveFcn=dspblkCoreblockFVToolHelper(gcbh,'postsave');  CloseFcn=dspblkCoreblockFVToolHelper(gcbh,'close');
  Discrete Transfer Fcn2 : DiscreteTransferFcn  LoadFcn=dspblkCoreblockFVToolHelper(gcbh,'load');  Numerator=[0.37152]  Denominator=[1 -.62848]
      settings: CopyFcn=dspblkCoreblockFVToolHelper(gcbh,'copy');  DeleteFcn=dspblkCoreblockFVToolHelper(gcbh,'close');  ModelCloseFcn=dspblkCoreblockFVToolHelper(gcbh,'close');  PreSaveFcn=dspblkCoreblockFVToolHelper(gcbh,'presave');  PostSaveFcn=dspblkCoreblockFVToolHelper(gcbh,'postsave');  CloseFcn=dspblkCoreblockFVToolHelper(gcbh,'close');
  Out1 : Outport
  wires:
  In1/1 -> Discrete Transfer Fcn2/1
  Discrete Transfer Fcn2/1 -> Out1/1

== system updated_target_driver_2026_withVariants_MPC_andwlqp/Variant Subsystem/Simulation/signal generator a3/Drive_Signal/FlattenedSine1 ==
  freq : Inport
  phase : Inport  Port=2
  a2 : Inport  Port=3
  0.1 : Gain  Gain=0.1
  1.1 : Gain  Gain=1.1
  2f : Gain  Gain=2
  2pi : Gain  Gain=2*pi
  3f : Gain  Gain=3
  Add : Sum  Inputs=+++
  Add1 : Sum
  Amplitude Correction : Subsystem  Commented=on
  AveragedAmp_filtered : Subsystem
  Product : Product
  first harmonic : Trigonometry  OutputSignalType=real
  integrate(omega*t) : DiscreteIntegrator  SampleTime=-1  ICPrevOutput=DiscIntNeverNeededParam  ICPrevScaledInput=DiscIntNeverNeededParam
  second harmonic : Trigonometry  OutputSignalType=real
  third harmonic : Trigonometry  OutputSignalType=real
  split cycle signal : Outport
  wires:
  freq/1 -> 2pi/1
  2pi/1 -> integrate(omega*t)/1
  3f/1 -> third harmonic/1
  first harmonic/1 -> 1.1/1
  third harmonic/1 -> 0.1/1
  1.1/1 -> Add/1
  Add1/1 -> first harmonic/1, 2f/1, 3f/1
  integrate(omega*t)/1 -> Add1/1
  phase/1 -> Add1/2
  2f/1 -> second harmonic/1
  0.1/1 -> Add/2
  Product/1 -> Add/3
  second harmonic/1 -> Product/1
  Add/1 -> split cycle signal/1
  a2/1 -> AveragedAmp_filtered/1(In1)
  AveragedAmp_filtered/1(Out1) -> Product/2

== system updated_target_driver_2026_withVariants_MPC_andwlqp/Variant Subsystem/Simulation/signal generator a3/Drive_Signal/FlattenedSine_phase ==
  f : Inport
  phase : Inport  Port=2
  0.1 : Gain  Gain=0.1
  1.1 : Gain  Gain=1.1
  2pi : Gain  Gain=2*pi
  3f : Gain  Gain=3
  Add : Sum
  Sum : Sum  Inputs=|++
  first harmonic : Trigonometry  OutputSignalType=real
  integrate(omega*t) : DiscreteIntegrator  SampleTime=-1  ICPrevOutput=DiscIntNeverNeededParam  ICPrevScaledInput=DiscIntNeverNeededParam
  pi/180 : Gain  Gain=pi/180
  third harmonic : Trigonometry  OutputSignalType=real
  split cycle signal : Outport
  wires:
  f/1 -> 2pi/1
  2pi/1 -> integrate(omega*t)/1
  3f/1 -> third harmonic/1
  first harmonic/1 -> 1.1/1
  third harmonic/1 -> 0.1/1
  1.1/1 -> Add/1
  0.1/1 -> Add/2
  Add/1 -> split cycle signal/1
  Sum/1 -> first harmonic/1, 3f/1
  pi/180/1 -> Sum/2
  integrate(omega*t)/1 -> Sum/1
  phase/1 -> pi/180/1

== system updated_target_driver_2026_withVariants_MPC_andwlqp/Variant Subsystem/Simulation/signal generator a3/Drive_Signal/SignalForRamp_binary ==
  note: Should output 1 or -1,
      | so signal ramps UP to 1
      | or DOWN to 0.
  In1 : Inport
  Add : Sum  Inputs=+-
  Compare To Zero : simulink/Logic and Bit Operations/Compare To Zero  relop=>  OutDataTypeStr=uint8  ZeroCross=off
  Constant : Constant
  Data Type Conversion : DataTypeConversion  OutDataTypeStr=double  SaturateOnIntegerOverflow=off  RndMeth=Floor
  Gain : Gain  Gain=2
  Out1 : Outport
  wires:
  In1/1 -> Compare To Zero/1
  Compare To Zero/1 -> Data Type Conversion/1
  Gain/1 -> Add/1
  Constant/1 -> Add/2
  Add/1 -> Out1/1
  Data Type Conversion/1 -> Gain/1

== system updated_target_driver_2026_withVariants_MPC_andwlqp/Variant Subsystem/Simulation/signal generator a3/Drive_Signal/SignalForSin_binary ==
  note: We want this to stay "high" for 1
      | second after the actual "enable"
      | is turned off...
  In1 : Inport
  Compare To Zero : simulink/Logic and Bit Operations/Compare To Zero  relop=>  OutDataTypeStr=uint8  ZeroCross=off
  Data Type Conversion : DataTypeConversion  OutDataTypeStr=double  SaturateOnIntegerOverflow=off  RndMeth=Floor
  Out1 : Outport
  wires:
  In1/1 -> Compare To Zero/1
  Compare To Zero/1 -> Data Type Conversion/1
  Data Type Conversion/1 -> Out1/1

== system updated_target_driver_2026_withVariants_MPC_andwlqp/Variant Subsystem/Simulation/signal generator a3/Drive_Signal/Sinewave ==
  In2 : Inport
  2pi : Gain  Gain=2*pi
  first harmonic : Trigonometry  OutputSignalType=real
  integrate(omega*t) : DiscreteIntegrator  SampleTime=-1  ICPrevOutput=DiscIntNeverNeededParam  ICPrevScaledInput=DiscIntNeverNeededParam
  split cycle signal : Outport
  wires:
  In2/1 -> 2pi/1
  2pi/1 -> integrate(omega*t)/1
  integrate(omega*t)/1 -> first harmonic/1
  first harmonic/1 -> split cycle signal/1

== system updated_target_driver_2026_withVariants_MPC_andwlqp/Variant Subsystem/Simulation/signal generator a3/Drive_Signal1/AveragedAmp_filtered ==
  note: To avoid having signal "jump",
      | we want SMOOTH transitions
      | in frequency (i.e., a weighted sum
      | of current freq and freq some delta t ago)
  note: time constant 0.002sec
      | for 10kHz samping
  In1 : Inport
  Discrete Transfer Fcn1 : DiscreteTransferFcn  LoadFcn=dspblkCoreblockFVToolHelper(gcbh,'load');  Numerator=[0.05]  Denominator=[1 -.95]
      settings: CopyFcn=dspblkCoreblockFVToolHelper(gcbh,'copy');  DeleteFcn=dspblkCoreblockFVToolHelper(gcbh,'close');  ModelCloseFcn=dspblkCoreblockFVToolHelper(gcbh,'close');  PreSaveFcn=dspblkCoreblockFVToolHelper(gcbh,'presave');  PostSaveFcn=dspblkCoreblockFVToolHelper(gcbh,'postsave');  CloseFcn=dspblkCoreblockFVToolHelper(gcbh,'close');
  Discrete Transfer Fcn2 : DiscreteTransferFcn  LoadFcn=dspblkCoreblockFVToolHelper(gcbh,'load');  Numerator=[0.37152]  Denominator=[1 -.62848]
      settings: CopyFcn=dspblkCoreblockFVToolHelper(gcbh,'copy');  DeleteFcn=dspblkCoreblockFVToolHelper(gcbh,'close');  ModelCloseFcn=dspblkCoreblockFVToolHelper(gcbh,'close');  PreSaveFcn=dspblkCoreblockFVToolHelper(gcbh,'presave');  PostSaveFcn=dspblkCoreblockFVToolHelper(gcbh,'postsave');  CloseFcn=dspblkCoreblockFVToolHelper(gcbh,'close');
  Out1 : Outport
  wires:
  In1/1 -> Discrete Transfer Fcn2/1
  Discrete Transfer Fcn2/1 -> Out1/1
